simulink model "overload_controller"  (R2021b)
settings: Solver=VariableStepAuto  StartTime=0.0  StopTime=10.0  RelTol=1e-3
settings Model: Creator=aoa  LastModifiedBy=aoa

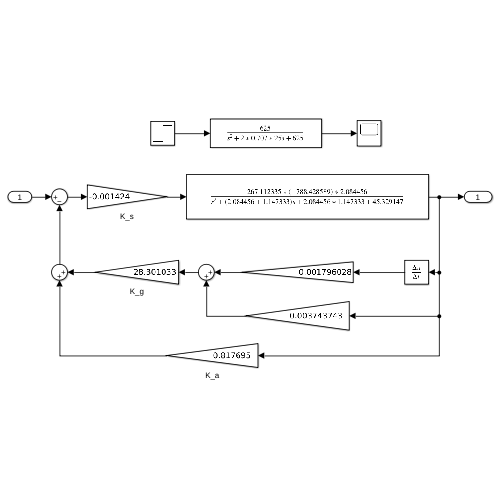
[thumbnail: Simulink's stored preview of the top-level diagram]
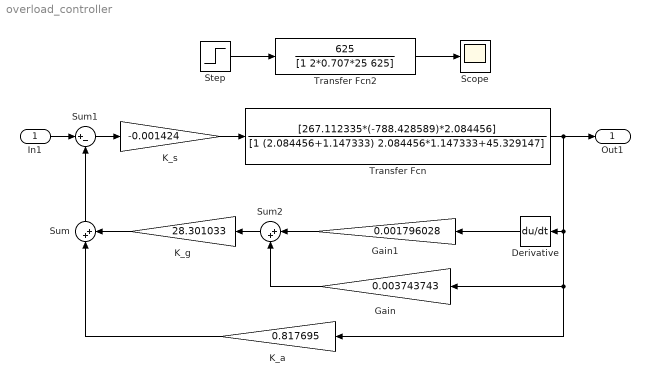
== system overload_controller ==
  In1 : Inport
  Derivative : Derivative  CoefficientInTFapproximation=0.0000000001
  Gain : Gain  Gain=0.003743743
  Gain1 : Gain  Gain=0.001796028
  K_a : Gain  Gain=0.817695
  K_g : Gain  Gain=28.301033
  K_s : Gain  Gain=-0.001424
  Scope : Scope
  Step : Step  SampleTime=0
  Sum : Sum  Inputs=|++
  Sum1 : Sum  Inputs=|+-
  Sum2 : Sum  Inputs=|++
  Transfer Fcn : TransferFcn  Numerator=[267.112335*(-788.428589)*2.084456]  Denominator=[1 (2.084456+1.147333) 2.084456*1.147333+45.329147]
  Transfer Fcn2 : TransferFcn  Numerator=[625]  Denominator=[1 2*0.707*25 625]
  Out1 : Outport
  wires:
  Sum1/1 -> K_s/1
  K_s/1 -> Transfer Fcn/1
  Transfer Fcn/1 -> Out1/1, Derivative/1, Gain/1, K_a/1
  K_g/1 -> Sum/2
  Sum/1 -> Sum1/2
  K_a/1 -> Sum/1
  Sum2/1 -> K_g/1
  Derivative/1 -> Gain1/1
  Gain/1 -> Sum2/2
  Gain1/1 -> Sum2/1
  In1/1 -> Sum1/1
  Step/1 -> Transfer Fcn2/1
  Transfer Fcn2/1 -> Scope/1
